simulink model "model_simulink_PI"  (R2022b)
settings: Solver=VariableStepAuto  StartTime=0.0  StopTime=600  FixedStep=0.5  RelTol=1e-3
values from neighbouring files (symbols this model uses):
  K = 10.6    [init.m]
  m_offset = 24.71    [init.m]
  T = 340    [init.m]
  T_o = 10    [init.m]
  y_ref = 28    [init.m]
settings Model: Creator=mikolaj  LastModifiedBy=mikolaj

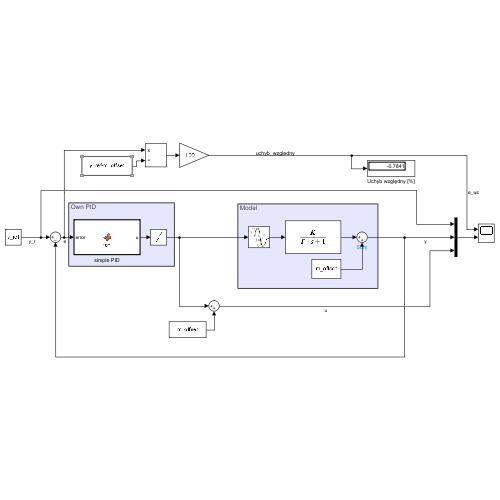
[thumbnail: Simulink's stored preview of the top-level diagram]
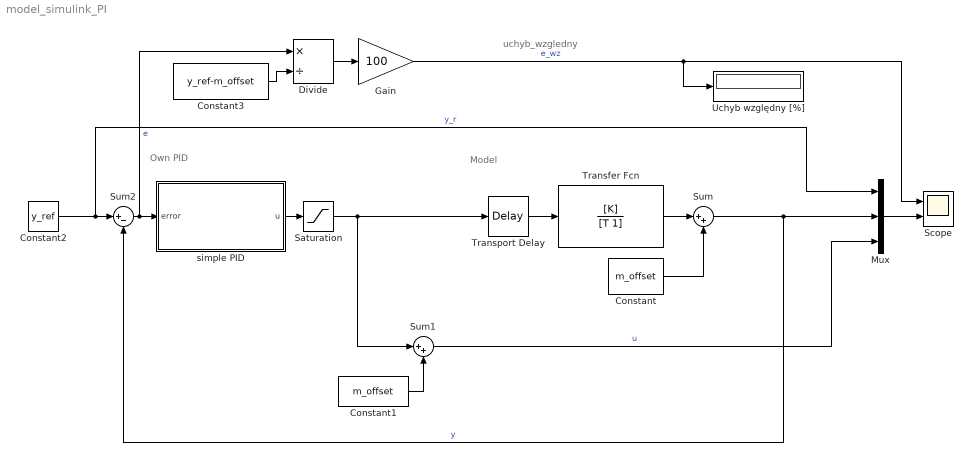
== system model_simulink_PI ==
  note: uchyb_wzgledny
  note: Own PID
  note: Model
  Constant : Constant  Value=m_offset
  Constant1 : Constant  Value=m_offset
  Constant2 : Constant  Value=y_ref
  Constant3 : Constant  Value=y_ref-m_offset
  Divide : Product  Inputs=*/  RndMeth=Zero  SaturateOnIntegerOverflow=on
  Gain : Gain  Gain=100
  Mux : Mux  Inputs=3
  Saturation : Saturate  UpperLimit=1  LowerLimit=0
  Scope : Scope  NumInputPorts=2
  Sum : Sum  Inputs=|++
  Sum1 : Sum  Inputs=|++
  Sum2 : Sum  Inputs=|+-
  Transfer Fcn : TransferFcn  Numerator=[K]  Denominator=[T 1]
  Transport Delay : TransportDelay  DelayTime=T_o
  Uchyb względny [%] : Display
  simple PID : MATLAB Function  TreatAsAtomicUnit=on
  wires:
  Transport Delay/1 -> Transfer Fcn/1
  Constant/1 -> Sum/2
  Transfer Fcn/1 -> Sum/1
  simple PID/1(u) -> Saturation/1
  Saturation/1 -> Sum1/1, Transport Delay/1
  Constant1/1 -> Sum1/2
  Sum2/1 -> Divide/1, simple PID/1(error)  "e"
  Sum/1 -> Sum2/2, Mux/2  "y"
  Sum1/1 -> Mux/3  "u"
  Constant2/1 -> Mux/1, Sum2/1  "y_r"
  Mux/1 -> Scope/2
  Constant3/1 -> Divide/2
  Divide/1 -> Gain/1
  Gain/1 -> Uchyb względny [%]/1, Scope/1  "e_wz"

== matlab function model_simulink_PI/simple PID ==
  settings: updateMethod=DISCRETE
  data: error input; u output
function u = fcn(error)

persistent previous_error;
if isempty(previous_error)
    previous_error = 0;
end

persistent previous_integral;
if isempty(previous_integral)
    previous_integral = 0;
end

% parameters
dt = 1;
k_p = 2.2;
k_i = 0.002;
k_d = 0;

% proportional part
u_P = k_p * error;

% integral part
integral = previous_integral + (error + previous_error);
previous_integral = integral;
u_I = k_i * integral * (dt/2);

% derivative part
derivative = (error - previous_error)/dt;
previous_error = error;
u_D = k_d * derivative;

% sum
u = u_P + u_I + u_D;
